simulink model "quydaomain"  (R2015a)
settings: Solver=ode45  StartTime=0.0  StopTime=322  RelTol=1e-3
settings Model: Creator=Roronoa zoro  LastModifiedBy=Administrator

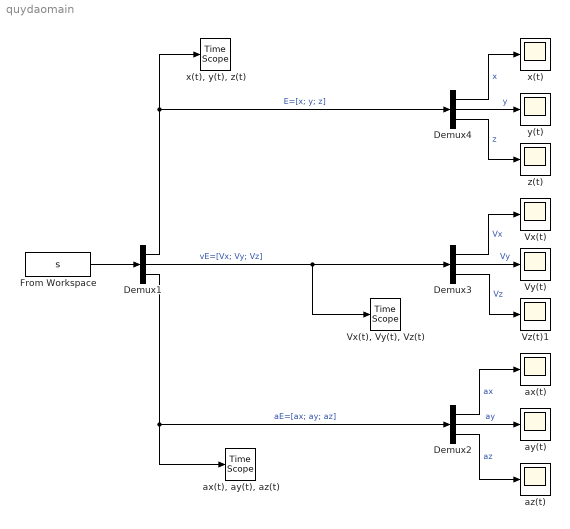
== system quydaomain ==
  Demux{1..4} (4 alike) : Demux  Outputs=3
  From Workspace : FromWorkspace  VariableName=s  SampleTime=0.08
  Vx(t) : Scope
      settings: SaveName=ScopeData6
  "Vx(t), Vy(t), Vz(t)" : TimeScope
  Vy(t) : Scope
      settings: SaveName=ScopeData7
  Vz(t)1 : Scope
      settings: YMax=20  SaveName=ScopeData8  SampleInput=on
  ax(t) : Scope
      settings: SaveName=ScopeData9
  "ax(t), ay(t), az(t)" : TimeScope
  ay(t) : Scope
      settings: SaveName=ScopeData10
  az(t) : Scope
      settings: SaveName=ScopeData11
  x(t) : Scope
      settings: SaveName=ScopeData3  ScrollMode=on
  "x(t), y(t), z(t)" : TimeScope
  y(t) : Scope
      settings: SaveName=ScopeData4
  z(t) : Scope
      settings: SaveName=ScopeData5
  wires:
  From Workspace/1 -> Demux1/1
  Demux1/1 -> "x(t), y(t), z(t)"/1, Demux4/1  "E=[x; y; z]"
  Demux1/2 -> Demux3/1, "Vx(t), Vy(t), Vz(t)"/1  "vE=[Vx; Vy; Vz]"
  Demux1/3 -> "ax(t), ay(t), az(t)"/1, Demux2/1  "aE=[ax; ay; az]"
  Demux4/1 -> x(t)/1  "x"
  Demux4/2 -> y(t)/1  "y"
  Demux4/3 -> z(t)/1  "z"
  Demux3/1 -> Vx(t)/1  "Vx"
  Demux3/2 -> Vy(t)/1  "Vy"
  Demux3/3 -> Vz(t)1/1  "Vz"
  Demux2/1 -> ax(t)/1  "ax"
  Demux2/2 -> ay(t)/1  "ay"
  Demux2/3 -> az(t)/1  "az"
